simulink model "Code_Trafficlights"  (R2023b)
settings: Solver=FixedStepDiscrete  StartTime=0.0  StopTime=10.0  FixedStep=1e-3  RelTol=1e-3
settings Model: Creator=hp  LastModifiedBy=hp
settings SolverCC: AutoInsertRateTranBlk=on
settings OptimizationCC: DefaultParameterBehavior=Inlined  UseDivisionForNetSlopeComputation=on  GainParamInheritBuiltInType=on  UseFloatMulNetSlope=on  InlineInvariantSignals=on  PassReuseOutputArgsAs=Individual arguments  ZeroExternalMemoryAtStartup=off  ZeroInternalMemoryAtStartup=off  NoFixptDivByZeroProtection=on  EfficientFloat2IntCast=on  LifeSpan=1  OptimizeBlockOrder=speed  DifferentSizesBufferReuse=on  EfficientTunableParamExpr=on
settings DebuggingCC: ParameterTunabilityLossMsg=error
settings HardwareCC: ProdBitPerInt=16  ProdBitPerPointer=16  ProdBitPerSizeT=16  ProdBitPerPtrDiffT=16  ProdLargestAtomicFloat=None  ProdWordSize=8  ProdLongLongMode=on  ProdHWDeviceType=Atmel->AVR
settings SFSimCC: MATLABDynamicMemAlloc=off
settings RTWCC: Description=Embedded Coder  SystemTargetFile=ert.tlc  TemplateMakefile=ert_default_tmf
settings CodeAppCC: ForceParamTrailComments=on  IgnoreCustomStorageClasses=off  OperatorAnnotations=on  SimulinkDataObjDesc=on  SFDataObjDesc=on  CustomSymbolStrGlobalVar=rt$N$M  CustomSymbolStrType=$N$M  CustomSymbolStrFcn=$N$M$F  CustomSymbolStrMacro=$N$M  InsertBlockDesc=on
settings ERTTargetCC: TargetLangStandard=C99 (ISO)  GenerateSampleERTMain=on  IncludeMdlTerminateFcn=off  CombineSignalStateStructs=on  SupportAbsoluteTime=off  SupportComplex=off  SupportNonInlinedSFcns=on  InlinedParameterPlacement=NonHierarchical  ERTCustomFileTemplate=example_file_process.tlc  ERTFilePackagingFormat=CompactWithDataFile

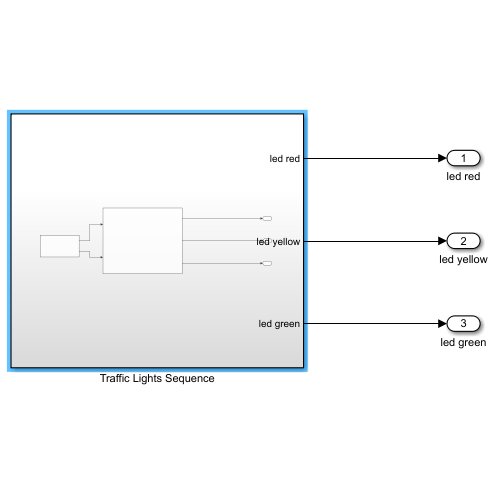
[thumbnail: Simulink's stored preview of the top-level diagram]
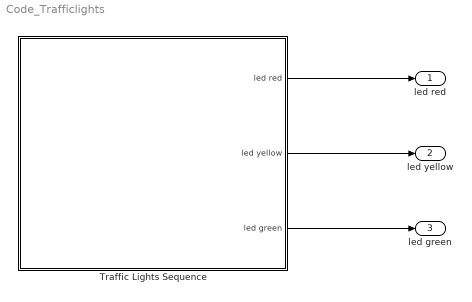
== system Code_Trafficlights ==
  Traffic Lights Sequence : Subsystem
  led red : Outport
  led yellow : Outport  Port=2
  led green : Outport  Port=3
  wires:
  Traffic Lights Sequence/1(led red) -> led red/1
  Traffic Lights Sequence/2(led yellow) -> led yellow/1
  Traffic Lights Sequence/3(led green) -> led green/1

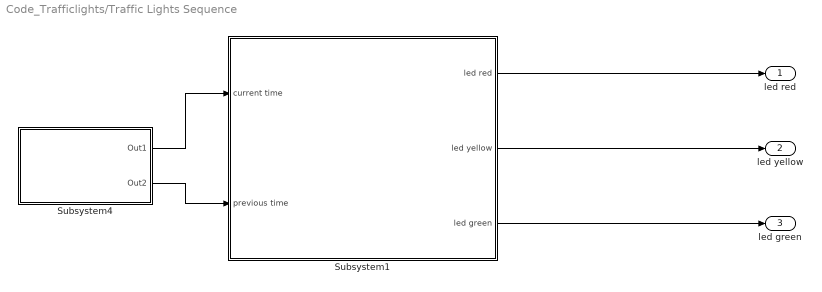
== system Code_Trafficlights/Traffic Lights Sequence ==
  Subsystem1 : Subsystem  TreatAsAtomicUnit=on
  Subsystem4 : Subsystem
  led red : Outport
  led yellow : Outport  Port=2
  led green : Outport  Port=3
  wires:
  Subsystem4/1(Out1) -> Subsystem1/1(current time)
  Subsystem4/2(Out2) -> Subsystem1/2(previous time)
  Subsystem1/1(led red) -> led red/1
  Subsystem1/3(led green) -> led green/1
  Subsystem1/2(led yellow) -> led yellow/1

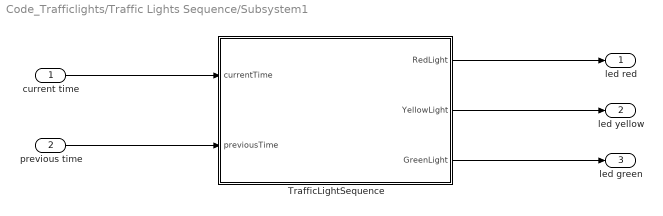
== system Code_Trafficlights/Traffic Lights Sequence/Subsystem1 ==
  current time : Inport
  previous time : Inport  Port=2
  TrafficLightSequence : MATLAB Function  TreatAsAtomicUnit=on
  led red : Outport
  led yellow : Outport  Port=2
  led green : Outport  Port=3
  wires:
  current time/1 -> TrafficLightSequence/1(currentTime)
  previous time/1 -> TrafficLightSequence/2(previousTime)
  TrafficLightSequence/1(RedLight) -> led red/1
  TrafficLightSequence/2(YellowLight) -> led yellow/1
  TrafficLightSequence/3(GreenLight) -> led green/1

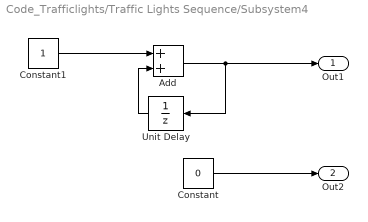
== system Code_Trafficlights/Traffic Lights Sequence/Subsystem4 ==
  Add : Sum
  Constant : Constant  Value=0
  Constant1 : Constant
  Unit Delay : UnitDelay  SampleTime=2  HasFrameUpgradeWarning=on
  Out1 : Outport
  Out2 : Outport  Port=2
  wires:
  Constant/1 -> Out2/1
  Add/1 -> Unit Delay/1, Out1/1
  Constant1/1 -> Add/1
  Unit Delay/1 -> Add/2

== matlab function Code_Trafficlights/Traffic Lights Sequence/Subsystem1/TrafficLightSequence ==
  data: currentTime input; RedLight output; previousTime input; YellowLight output; GreenLight output
function [RedLight, YellowLight, GreenLight] = TrafficLightSequenceContinuous(currentTime, previousTime)
    % Continuous traffic light sequence
    
    % Adjust timing parameters (in seconds)
    redTime = 2;     % Set the duration for the red light
    yellowTime = 2;   % Set the duration for the yellow light
    greenTime = 2;   % Set the duration for the green light

    % Initialize outputs
    RedLight = 0;
    YellowLight = 0;
    GreenLight = 0;

    % Calculate elapsed time since the last update
    elapsedTime = currentTime - previousTime;

    % Calculate the time within a complete cycle
    cycleTime = redTime + yellowTime + greenTime;

    % Determine the current phase in the cycle
    currentPhase = mod(elapsedTime, cycleTime);

    % Traffic light sequence logic
    if currentPhase < redTime
        % Red light is ON
        RedLight = 1;
    elseif currentPhase < redTime + yellowTime
        % Yellow light is ON
        YellowLight = 1;
    else
        % Green light is ON
        GreenLight = 1;
    end
end
